simulink model "cosim"  (Simulink 8.2)
settings: Solver=FixedStepDiscrete  SolverMode=SingleTasking  StartTime=0.0  StopTime=inf  FixedStep=0.01  RelTol=1e-3
undefined symbols (not defined in the file or in its folder): A, N
libraries: simulink x5, xbsIndex_r4 x1, JTAGRuntimeCosim_r4 x1
settings Model: Creator=gaborsz  LastModifiedBy=laca
settings DebuggingCC: FcnCallInpInsideContextMsg=EnableAllAsWarning
settings GRTTargetCC: CombineOutputUpdateFcns=on  GRTInterface=off

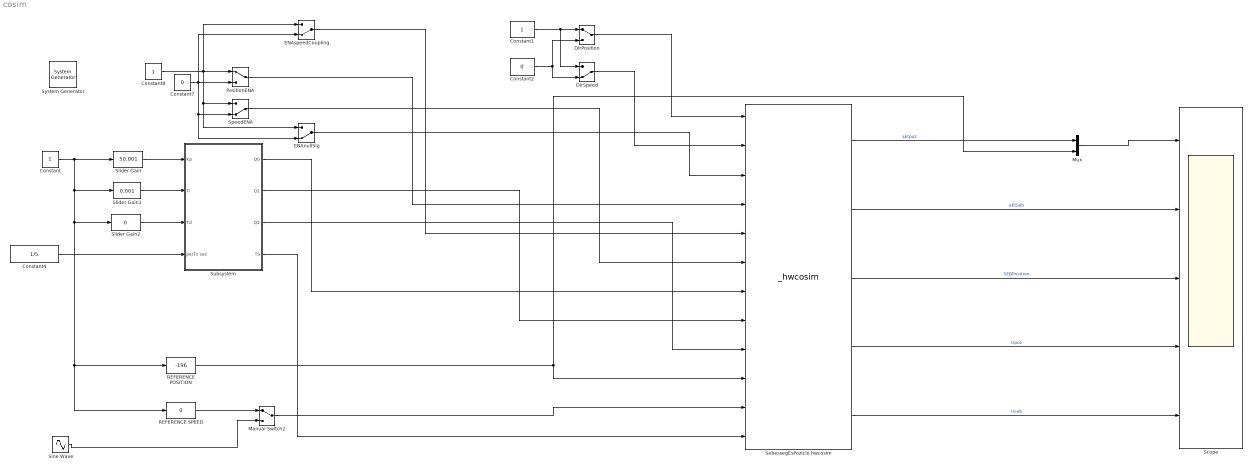
== system cosim ==
  " System Generator" : xbsIndex_r4/ System Generator  Tag=genX  xilinxfamily=spartan3e  part=xc3s500e  speed=-4  package=pq208  synthesis_tool=XST  clock_wrapper=Clock Enables  directory=./netlist  proj_type=Project Navigator  Synth_file=XST Defaults  Impl_file=ISE Defaults  testbench=off  simulink_period=1  sysclk_period=20  dcm_input_clock_period=10  incr_netlist=off  trim_vbits=Everywhere in SubSystem  dbl_ovrd=According to Block Masks  core_generation=According to Block Masks  run_coregen=off  deprecated_control=off  eval_field=0  block_type=sysgen
  Constant : Constant
  Constant1 : Constant
  Constant2 : Constant  Value=0
  Constant4 : Constant  Value=1/5
  Constant7 : Constant  Value=0
  Constant8 : Constant
  DirPosition : ManualSwitch
  DirSpeed : ManualSwitch  CurrentSetting=0
  ENAnullSig : ManualSwitch  CurrentSetting=0
  ENAspeedCoupling : ManualSwitch  CurrentSetting=0
  Manual Switch2 : ManualSwitch
  Mux : Mux  Inputs=2
  PositionENA : ManualSwitch
  REFERENCE POSITION : simulink/Math Operations/Slider Gain  low=-200  gain=-196  high=200
  REFERENCE SPEED : simulink/Math Operations/Slider Gain  low=-200  gain=0  high=200
  Scope : Scope  NumInputPorts=5
      settings: YMin=-250~-1~15~65000~-1  YMax=2000~1~37.5~65000~1
  SebessegEsPozicio hwcosim : JTAGRuntimeCosim_r4/_hwcosim  clkSrc=Free Running  hasCombinationalPath=off  bitfileName=C:\Diak\gl\SPARTAN3E500K_slave\SystemGenrator\SebessegEsPozicio\netlist\sebessegespozicio_cw.bit  skipConfig=off  cable=Auto Detect  speed=N/A  cablePort=N/A  cableLocation=Local  shareCable=off  enable_codebug=on  design_xtable=|  engineDll=JTAGCosimEngine.dll  cableWaitTime=10  bscanPos=1  IRLengths=[6,8]  useWaitBox=1  hasBufgmux=on  Scheme=Cosim  useCmdProc=1  hasProc=0  useImpact=0  printLogFile=0  block_type=jtagcosim
      | {
      |   'clkWrapper' => 'sebessegespozicio_cw',
      |   'clocksGcd' => undef,
      |   'device' => 'xc3s500e-4pq208',
      |   'ports' => {
      |     'aktpoz' => {
      |       'bd_port_index' => 0,
      |       'direction' => 'out',
      |       'icon_text' => 'aktpoz',
      |       'period' => 1,
      |       'sim_pause_trigger' => false,
      |       'type' => 'Fix_16_0',
      |       'width' => 16,
      |     },
      |     'aktseb' => {
      |       'bd_port_index' => 1,
      |       'direction' => 'out',
      |       'icon_text' => 'aktSeb',
      |       'period' => 1,
      |       'sim_pause_trigger' => false,
      |       'type' => 'Fix_16_0',
      |       'width' => 16,
      |     },
      |     'csere_poz' => {
      |       'bd_port_index' => 0,
      |       'direction' => 'in',
      |       'icon_text' => 'CSere_poz',
      |       'period' => 1,
      |       'sim_pause_trigger' => false,
      |       'type' => 'Bool',
      |       'width' => 1,
      |     },
      |     'csere_seb' => {
      |       'bd_port_index' => 1,
      |       'direction' => 'in',
      |       'icon_text' => 'CSere_seb',
      |       'period' => 1,
      |       'sim_pause_trigger' => false,
      |       'type' => 'Bool',
      |       'width' => 1,
      |     },
      |     'enanullsigposition' => {
      |       'bd_port_index' => 2,
      |       'direction' => 'in',
      |       'icon_text' => 'EnaNullSigPosition',
      |       'period' => 1,
      |       'sim_pause_trigger' => false,
      |       'type' => 'Bool',
      |       'width' => 1,
      |     },
      |     'enapositionpwm' => {
      |       'bd_port_index' => 3,
      |       'direction' => 'in',
      |       'icon_text' => 'EnaPositionPwm',
      |       'period' => 1,
      |       'sim_pause_trigger' => false,
      |       'type' => 'Bool',
      |       'width' => 1,
      |     },
      |     'enaspeedcoupling' => {
      |       'bd_port_index' => 4,
      |       'direction' => 'in',
      |       'icon_text' => 'EnaSpeedCoupling',
      |       'period' => 1,
      |       'sim_pause_trigger' => false,
      |       'type' => 'Bool',
      |       'width' => 1,
      |     },
      |     'enaspeedpwm' => {
      |       'bd_port_index' => 5,
      |       'direction' => 'in',
      |       'icon_text' => 'EnaSpeedPwm',
      |       'period' => 1,
      |       'sim_pause_trigger' => false,
      |       'type' => 'Bool',
      |       'width' => 1,
      |     },
      |     'pozseb' => {
      |       'bd_port_index' => 2,
      |       'direction' => 'out',
      |       'icon_text' => 'PozSeb',
      |       'period' => 1,
      |       'sim_pause_trigger' => false,
      |       'type' => 'Fix_16_0',
      |       'width' => 16,
      |     },
      |     'q0' => {
      |       'bd_port_index' => 6,
      |       'direction' => 'in',
      |       'icon_text' => 'q0',
      |       'period' => 1,
      |       'sim_pause_trigger' => false,
      |       'type' => 'UFix_16_0',
      |       'width' => 16,
      |     },
      |     'q1' => {
      |       'bd_port_index' => 7,
      |       'direction' => 'in',
      |       'icon_text' => 'q1',
      |       'period' => 1,
      |       'sim_pause_trigger' => false,
      |       'type' => 'UFix_16_0',
      |       'width' => 16,
      |     },
      |     'q2' => {
      |       'bd_port_index' => 8,
      |       'direction' => 'in',
      |       'icon_text' => 'q2',
      |       'period' => 1,
      |       'sim_pause_trigger' => false,
      |       'type' => 'UFix_16_0',
      |       'width' => 16,
      |     },
      |     'refposition' => {
      |       'bd_port_index' => 9,
      |       'direction' => 'in',
      |       'icon_text' => 'refPosition',
      |       'period' => 1,
      |       'sim_pause_trigger' => false,
      |       'type' => 'Fix_16_0',
      |       'width' => 16,
      |     },
      |     'refspeed' => {
      |       'bd_port_index' => 10,
      |       'direction' => 'in',
      |       'icon_text' => 'refSpeed',
      |       'period' => 1,
      |       'sim_pause_trigger' => false,
      |       'type' => 'Fix_16_0',
      |       'width' => 16,
      |     },
      |     'tspid' => {
      |       'bd_port_index' => 11,
      |       'direction' => 'in',
      |       'icon_text' => 'TSpid',
      |       'period' => 1,
      |       'sim_pause_trigger' => false,
      |       'type' => 'UFix_32_0',
      |       'width' => 32,
      |     },
      |     'upoz' => {
      |       'bd_port_index' => 3,
      |       'direction' => 'out',
      |       'icon_text' => 'Upoz',
      |       'period' => 1,
      |       'sim_pause_trigger' => false,
      |       'type' => 'Fix_17_0',
      |       'width' => 17,
      |     },
      |     'useb' => {
      |       'bd_port_index' => 4,
      |       'direction' => 'out',
      |       'icon_text' => 'Useb',
      |       'period' => 1,
      |       'sim_pause_trigger' => false,
      |       'type' => 'Fix_17_0',
      |       'width' => 17,
      |     },
      |   },
      |   'shared_memories' => {},
      | }
  Sine Wave : Sin  Amplitude=90  Frequency=0.1  SampleTime=1
  Slider Gain : simulink/Math Operations/Slider Gain  low=0.001  gain=50.001  high=1300
  Slider Gain1 : simulink/Math Operations/Slider Gain  low=0  gain=0.001  high=10000000
  Slider Gain2 : simulink/Math Operations/Slider Gain  low=0  gain=0  high=5000
  SpeedENA : ManualSwitch  CurrentSetting=0
  Subsystem : Subsystem
  wires:
  Constant8/1 -> PositionENA/1, SpeedENA/1, ENAnullSig/1, ENAspeedCoupling/1
  Constant7/1 -> SpeedENA/2, ENAnullSig/2, ENAspeedCoupling/2, PositionENA/2
  Sine Wave/1 -> Manual Switch2/2
  REFERENCE SPEED/1 -> Manual Switch2/1
  Constant/1 -> Slider Gain/1, Slider Gain1/1, Slider Gain2/1, REFERENCE POSITION/1, REFERENCE SPEED/1
  Subsystem/2(Q1) -> SebessegEsPozicio hwcosim/8
  Subsystem/4(TS) -> SebessegEsPozicio hwcosim/12
  Slider Gain/1 -> Subsystem/1(Kp)
  Slider Gain1/1 -> Subsystem/2(Ti)
  Slider Gain2/1 -> Subsystem/3(Td)
  Constant4/1 -> Subsystem/4(perTs sec)
  Subsystem/1(Q0) -> SebessegEsPozicio hwcosim/7
  SpeedENA/1 -> SebessegEsPozicio hwcosim/6
  Manual Switch2/1 -> SebessegEsPozicio hwcosim/11
  SebessegEsPozicio hwcosim/2 -> Scope/2  "aktSeb"
  SebessegEsPozicio hwcosim/3 -> Scope/3  "SEBPosition"
  SebessegEsPozicio hwcosim/4 -> Scope/4  "Upoz"
  SebessegEsPozicio hwcosim/5 -> Scope/5  "Useb"
  Subsystem/3(Q2) -> SebessegEsPozicio hwcosim/9
  REFERENCE POSITION/1 -> SebessegEsPozicio hwcosim/10, Mux/2
  ENAnullSig/1 -> SebessegEsPozicio hwcosim/3
  PositionENA/1 -> SebessegEsPozicio hwcosim/4
  ENAspeedCoupling/1 -> SebessegEsPozicio hwcosim/5
  Constant1/1 -> DirSpeed/1, DirPosition/1
  Constant2/1 -> DirPosition/2, DirSpeed/2
  DirPosition/1 -> SebessegEsPozicio hwcosim/1
  DirSpeed/1 -> SebessegEsPozicio hwcosim/2
  Mux/1 -> Scope/1
  SebessegEsPozicio hwcosim/1 -> Mux/1  "aktpoz"

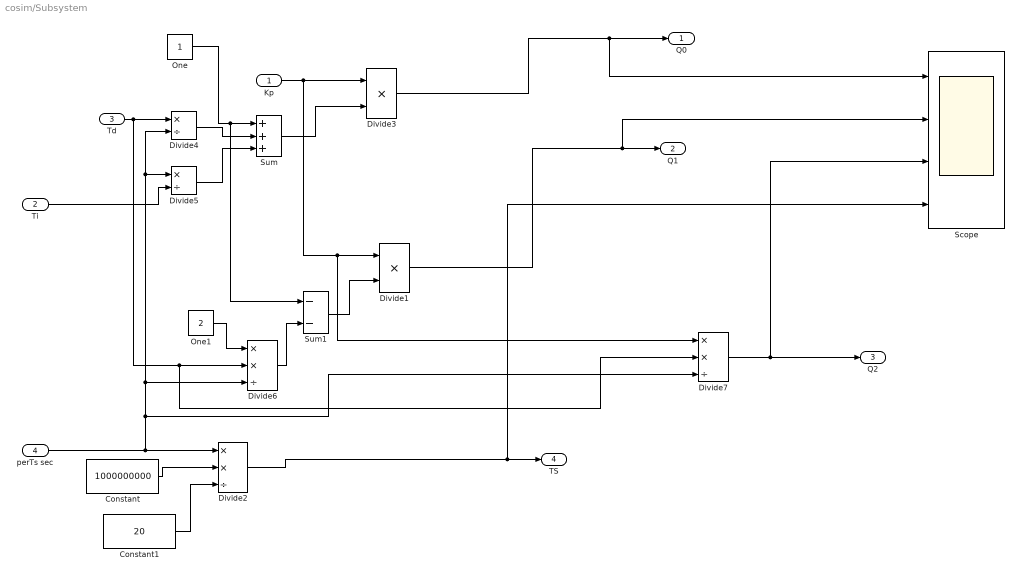
== system cosim/Subsystem ==
  Kp : Inport
  Ti : Inport  Port=2
  Td : Inport  Port=3
  perTs sec : Inport  Port=4
  Constant : Constant  Value=1000000000
  Constant1 : Constant  Value=20
  Divide1 : Product  Inputs=**
  Divide2 : Product  Inputs=**/
  Divide3 : Product  Inputs=**
  Divide4 : Product  Inputs=*/
  Divide5 : Product  Inputs=*/
  Divide6 : Product  Inputs=**/
  Divide7 : Product  Inputs=**/
  One : Constant
  One1 : Constant  Value=2
  Scope : Scope  NumInputPorts=4
      settings: YMin=2470.94~-2744.62~12.2932~9.5e+06  YMax=2731.04~-2483.22~13.5872~1.05e+07
  Sum : Sum  Inputs=+++
  Sum1 : Sum  Inputs=--
  Q0 : Outport
  Q1 : Outport  Port=2
  Q2 : Outport  Port=3
  TS : Outport  Port=4
  wires:
  Divide2/1 -> TS/1, Scope/4
  perTs sec/1 -> Divide2/1, Divide6/3, Divide4/2, Divide5/1, Divide7/3
  Constant/1 -> Divide2/2
  Constant1/1 -> Divide2/3
  Ti/1 -> Divide5/2
  Kp/1 -> Divide3/1, Divide1/1, Divide7/1
  Sum/1 -> Divide3/2
  Td/1 -> Divide4/1, Divide6/2, Divide7/2
  Divide5/1 -> Sum/3
  Divide4/1 -> Sum/2
  One/1 -> Sum/1, Sum1/1
  Divide3/1 -> Q0/1, Scope/1
  One1/1 -> Divide6/1
  Divide6/1 -> Sum1/2
  Sum1/1 -> Divide1/2
  Divide1/1 -> Q1/1, Scope/2
  Divide7/1 -> Q2/1, Scope/3
